simulink model "AM3"  (R2020b)
settings: Solver=VariableStepDiscrete  StartTime=0.0  StopTime=1.5e-3  MaxStep=1e-6  RelTol=1e-3
settings Model: Creator=seojoon  LastModifiedBy=seojoon

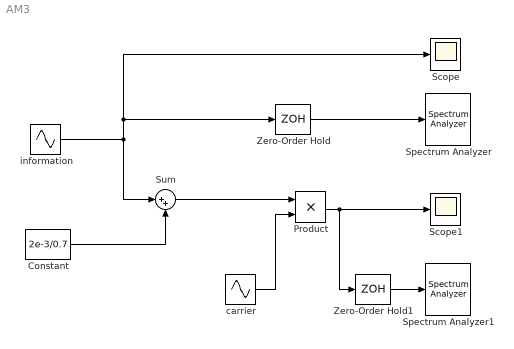
== system AM3 ==
  Constant : Constant  Value=2e-3/0.7  VectorParams1D=off
  Product : Product
  Scope : Scope
  Scope1 : Scope
  Spectrum Analyzer : SpectrumAnalyzer
  Spectrum Analyzer1 : SpectrumAnalyzer
  Sum : Sum  Inputs=|++
  Zero-Order Hold : ZeroOrderHold  SampleTime=(1.5e-3)/4096
  Zero-Order Hold1 : ZeroOrderHold  SampleTime=(1.5e-3)/4096
  carrier : Sin  Frequency=2*pi*700e3  Phase=pi/2  SampleTime=0
  information : Sin  Amplitude=2e-3  Frequency=2*pi*8000  SampleTime=0
  wires:
  information/1 -> Sum/1, Scope/1, Zero-Order Hold/1
  Constant/1 -> Sum/2
  Sum/1 -> Product/1
  carrier/1 -> Product/2
  Product/1 -> Zero-Order Hold1/1, Scope1/1
  Zero-Order Hold/1 -> Spectrum Analyzer/1
  Zero-Order Hold1/1 -> Spectrum Analyzer1/1
